simulink model "part2_2"  (R2018a)
settings: Solver=VariableStepAuto  StartTime=0.0  StopTime=10.0  MaxStep=0.01  RelTol=1e-3
settings Model: Creator=82354  LastModifiedBy=82354

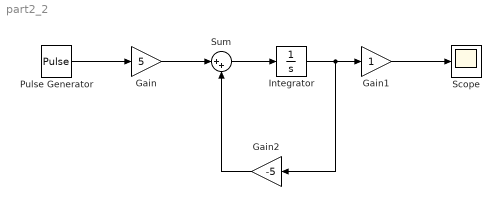
== system part2_2 ==
  Gain : Gain  Gain=5
  Gain1 : Gain
  Gain2 : Gain  Gain=-5
  Integrator : Integrator
  Pulse Generator : DiscretePulseGenerator  PulseType=Time based  Period=20  PulseWidth=5
  Scope : Scope
  Sum : Sum  Inputs=|++
  wires:
  Gain/1 -> Sum/1
  Pulse Generator/1 -> Gain/1
  Sum/1 -> Integrator/1
  Integrator/1 -> Gain2/1, Gain1/1
  Gain2/1 -> Sum/2
  Gain1/1 -> Scope/1
